simulink model "untitled1"  (R2023a)
settings: Solver=VariableStepAuto  StartTime=0.0  StopTime=10.0  RelTol=1e-3
values from neighbouring files (symbols this model uses):
  A = [0 1 0 0 ... (first row only)    [invpendulum.m]
  B = [0; -(1/M*L); 0; 1/M]    [invpendulum.m]
  C = eye(4)    [invpendulum.m]
  D = [0; 0; 0; 0]    [invpendulum.m]
  F = -acker(A, B, poles_desired)    [invpendulum.m]
  x_0 = [0.1; 0; 0.1; 0]    [invpendulum.m]
settings Model: Creator=ioloizou  LastModifiedBy=ioloizou

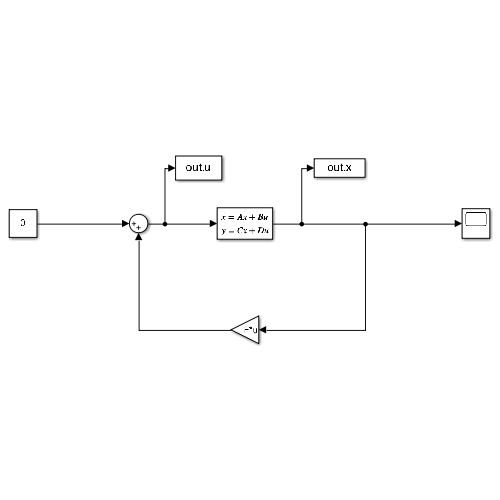
[thumbnail: Simulink's stored preview of the top-level diagram]
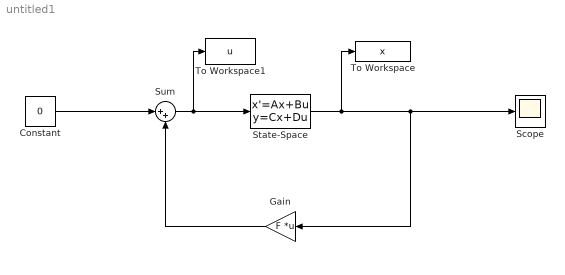
== system untitled1 ==
  Constant : Constant  Value=0
  Gain : Gain  Gain=F  Multiplication=Matrix(K*u)
  Scope : Scope
  State-Space : StateSpace  A=A  B=B  C=C  D=D  InitialCondition=x_0
  Sum : Sum  Inputs=|++
  To Workspace : ToWorkspace  VariableName=x  SampleTime=-1
      settings: Save2DSignal=2-D array (concatenate along first dimension)
  To Workspace1 : ToWorkspace  VariableName=u  SampleTime=-1
      settings: Save2DSignal=2-D array (concatenate along first dimension)
  wires:
  Constant/1 -> Sum/1
  Sum/1 -> To Workspace1/1, State-Space/1
  State-Space/1 -> To Workspace/1, Scope/1, Gain/1
  Gain/1 -> Sum/2
